simulink model "11_STATES_MBC_CPC"  (R2017b)
settings: Solver=VariableStepAuto  StartTime=0.0  StopTime=TMax  RelTol=1e-3
values from neighbouring files (symbols this model uses):
  alpha = exp(-2*pi*DT*fc)    [control_11_states_MBC_CPC.m]
  Dbar = zeros(size(Gbar,1),size(Kbar',2))    [control_11_states_MBC_CPC.m]
  DT = 0.01    [control_11_states_MBC_CPC.m]
  Gbar = [G 4*Gd]    [control_11_states_MBC_CPC.m]
  Lbar = (Abar + Bbar*Gbar - Kbar'*Cbar)    [control_11_states_MBC_CPC.m]
  PC_MaxPit = 1.570796    [control_11_states_MBC_CPC.m]
  PC_MaxRat = 0.1396263    [control_11_states_MBC_CPC.m]
  PC_MinPit = 0.0    (= 0)    [control_11_states_MBC_CPC.m]
  ref_pitch = 7.13132E-02    (= 0.0713132)    [control_11_states_MBC_CPC.m]
  ref_rot = 1.266999999999998    (= 1.267)    [control_11_states_MBC_CPC.m]
undefined symbols (not defined in the file or in its folder): OutList, strmatch
settings Model: Creator=Avell 1513  LastModifiedBy=Avell 1513

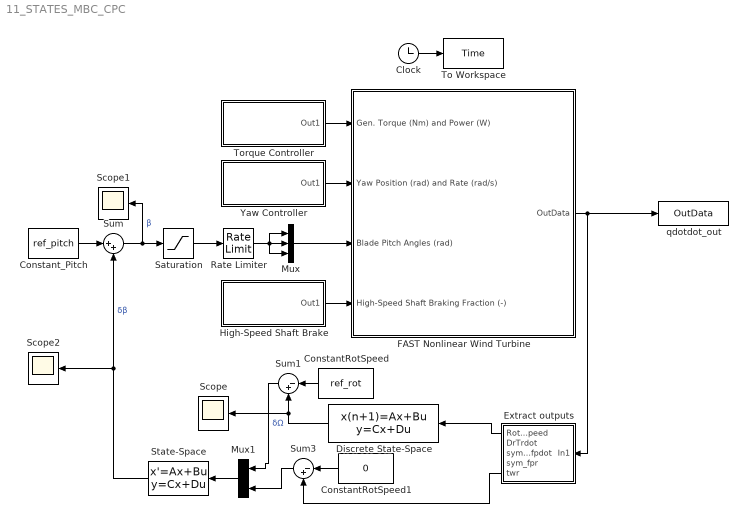
== system 11_STATES_MBC_CPC ==
  Clock : Clock
  ConstantRotSpeed : Constant  Value=ref_rot
  ConstantRotSpeed1 : Constant  Value=0
  Constant_Pitch : Constant  Value=ref_pitch
  Discrete State-Space : DiscreteStateSpace  A=alpha  B=1-alpha  C=alpha  D=1-alpha  InitialCondition=ref_rot  SampleTime=DT
  Extract outputs : Subsystem
  FAST Nonlinear Wind Turbine : Subsystem  mask(FAST Nonlinear Wind Turbine){}
      mask help: This block contains the FAST S-Function.
      mask init:
      | clear FAST_SFunc
  High-Speed Shaft Brake : Subsystem
  Mux : Mux  Inputs=3
  Mux1 : Mux  Inputs=2
  Rate Limiter : RateLimiter  RisingSlewLimit=PC_MaxRat  FallingSlewLimit=-PC_MaxRat  SampleTimeMode=inherited
  Saturation : Saturate  UpperLimit=PC_MaxPit  LowerLimit=PC_MinPit
  Scope : Scope
  Scope1 : Scope
  Scope2 : Scope
  State-Space : StateSpace  A=Lbar  B=Kbar'  C=Gbar  D=Dbar  InitialCondition=0
  Sum : Sum  Inputs=|++
  Sum1 : Sum  Inputs=|-+
  Sum3 : Sum  Inputs=|-+
  To Workspace : ToWorkspace  VariableName=Time  SampleTime=-1
  Torque Controller : Subsystem
  Yaw Controller : Subsystem
  qdotdot_out : ToWorkspace  VariableName=OutData  SampleTime=-1
  wires:
  State-Space/1 -> Sum/2, Scope2/1  "δβ"
  Yaw Controller/1(Out1) -> FAST Nonlinear Wind Turbine/2(Yaw Position (rad) and Rate (rad/s))
  High-Speed Shaft Brake/1(Out1) -> FAST Nonlinear Wind Turbine/4(High-Speed Shaft Braking Fraction (-))
  Discrete State-Space/1 -> Sum1/2, Scope/1
  Constant_Pitch/1 -> Sum/1
  FAST Nonlinear Wind Turbine/1(OutData) -> qdotdot_out/1, Extract outputs/1(In1)
  Saturation/1 -> Rate Limiter/1
  Clock/1 -> To Workspace/1
  Sum/1 -> Saturation/1, Scope1/1  "β"
  Rate Limiter/1 -> Mux/1, Mux/3, Mux/2
  ConstantRotSpeed/1 -> Sum1/1
  Mux/1 -> FAST Nonlinear Wind Turbine/3(Blade Pitch Angles (rad))
  Torque Controller/1(Out1) -> FAST Nonlinear Wind Turbine/1(Gen. Torque (Nm) and Power (W))
  Extract outputs/1(Rot_speed) -> Discrete State-Space/1
  Sum1/1 -> Mux1/1  "δΩ"
  Extract outputs/5(twr) -> Sum3/2
  Mux1/1 -> State-Space/1
  ConstantRotSpeed1/1 -> Sum3/1
  Sum3/1 -> Mux1/2

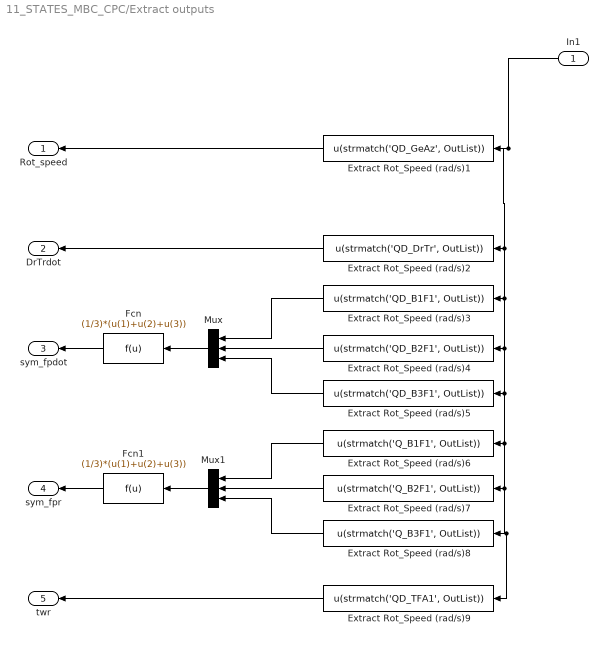
== system 11_STATES_MBC_CPC/Extract outputs ==
  In1 : Inport
  Extract Rot_Speed (rad/s)1 : Fcn  Expr=u(strmatch('QD_GeAz', OutList))
  Extract Rot_Speed (rad/s)2 : Fcn  Expr=u(strmatch('QD_DrTr', OutList))
  Extract Rot_Speed (rad/s)3 : Fcn  Expr=u(strmatch('QD_B1F1', OutList))
  Extract Rot_Speed (rad/s)4 : Fcn  Expr=u(strmatch('QD_B2F1', OutList))
  Extract Rot_Speed (rad/s)5 : Fcn  Expr=u(strmatch('QD_B3F1', OutList))
  Extract Rot_Speed (rad/s)6 : Fcn  Expr=u(strmatch('Q_B1F1', OutList))
  Extract Rot_Speed (rad/s)7 : Fcn  Expr=u(strmatch('Q_B2F1', OutList))
  Extract Rot_Speed (rad/s)8 : Fcn  Expr=u(strmatch('Q_B3F1', OutList))
  Extract Rot_Speed (rad/s)9 : Fcn  Expr=u(strmatch('QD_TFA1', OutList))
  Fcn : Fcn  Expr=(1/3)*(u(1)+u(2)+u(3))
  Fcn1 : Fcn  Expr=(1/3)*(u(1)+u(2)+u(3))
  Mux : Mux  Inputs=3
  Mux1 : Mux  Inputs=3
  Rot_speed : Outport
  DrTrdot : Outport  Port=2
  sym_fpdot : Outport  Port=3
  sym_fpr : Outport  Port=4
  twr : Outport  Port=5
  wires:
  Extract Rot_Speed (rad/s)1/1 -> Rot_speed/1
  Extract Rot_Speed (rad/s)2/1 -> DrTrdot/1
  In1/1 -> Extract Rot_Speed (rad/s)2/1, Extract Rot_Speed (rad/s)3/1, Extract Rot_Speed (rad/s)4/1, Extract Rot_Speed (rad/s)6/1, Extract Rot_Speed (rad/s)7/1, Extract Rot_Speed (rad/s)9/1, Extract Rot_Speed (rad/s)8/1, Extract Rot_Speed (rad/s)5/1, Extract Rot_Speed (rad/s)1/1
  Fcn/1 -> sym_fpdot/1
  Fcn1/1 -> sym_fpr/1
  Mux1/1 -> Fcn1/1
  Mux/1 -> Fcn/1
  Extract Rot_Speed (rad/s)3/1 -> Mux/1
  Extract Rot_Speed (rad/s)4/1 -> Mux/2
  Extract Rot_Speed (rad/s)5/1 -> Mux/3
  Extract Rot_Speed (rad/s)6/1 -> Mux1/1
  Extract Rot_Speed (rad/s)7/1 -> Mux1/2
  Extract Rot_Speed (rad/s)8/1 -> Mux1/3
  Extract Rot_Speed (rad/s)9/1 -> twr/1

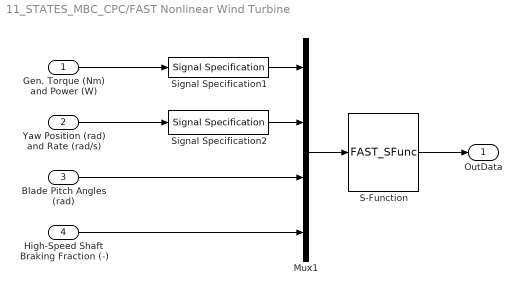
== system 11_STATES_MBC_CPC/FAST Nonlinear Wind Turbine ==
  Gen. Torque (Nm) and Power (W) : Inport
  Yaw Position (rad) and Rate (rad/s) : Inport  Port=2
  Blade Pitch Angles (rad) : Inport  Port=3
  High-Speed Shaft Braking Fraction (-) : Inport  Port=4
  Mux1 : Mux
  S-Function : S-Function  FunctionName=FAST_SFunc  Parameters=FAST_InputFileName, TMax, 0  SFunctionDeploymentMode=off  EnableBusSupport=off
  Signal Specification1 : SignalSpecification  OutDataTypeStr=double  Dimensions=2
  Signal Specification2 : SignalSpecification  OutDataTypeStr=double  Dimensions=2
  OutData : Outport
  wires:
  Gen. Torque (Nm) and Power (W)/1 -> Signal Specification1/1
  S-Function/1 -> OutData/1
  Mux1/1 -> S-Function/1
  Blade Pitch Angles (rad)/1 -> Mux1/3
  Yaw Position (rad) and Rate (rad/s)/1 -> Signal Specification2/1
  Signal Specification1/1 -> Mux1/1
  Signal Specification2/1 -> Mux1/2
  High-Speed Shaft Braking Fraction (-)/1 -> Mux1/4

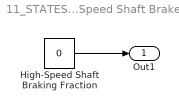
== system 11_STATES_MBC_CPC/High-Speed Shaft Brake ==
  High-Speed Shaft Braking Fraction : Constant  Value=0
  Out1 : Outport
  wires:
  High-Speed Shaft Braking Fraction/1 -> Out1/1

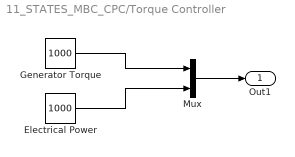
== system 11_STATES_MBC_CPC/Torque Controller ==
  Electrical Power : Constant  Value=1000
  Generator Torque : Constant  Value=1000
  Mux : Mux  Inputs=2
  Out1 : Outport
  wires:
  Mux/1 -> Out1/1
  Generator Torque/1 -> Mux/1
  Electrical Power/1 -> Mux/2

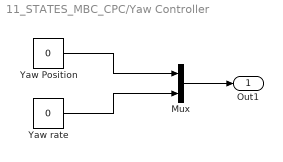
== system 11_STATES_MBC_CPC/Yaw Controller ==
  Mux : Mux  Inputs=2
  Yaw Position : Constant  Value=0
  Yaw rate : Constant  Value=0
  Out1 : Outport
  wires:
  Mux/1 -> Out1/1
  Yaw Position/1 -> Mux/1
  Yaw rate/1 -> Mux/2
